simulink model "gnc"  (R2023b)
settings: Solver=VariableStepAuto  StartTime=0.0  StopTime=10.0  RelTol=1e-3
settings Model: DataDictionary=gnc_private.sldd  EnableAccessToBaseWorkspace=off  Creator=Miguel  LastModifiedBy=Miguel

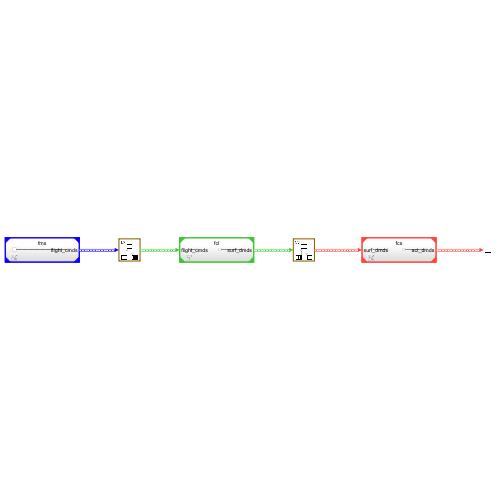
[thumbnail: Simulink's stored preview of the top-level diagram]
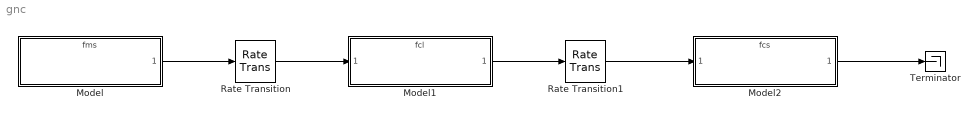
== system gnc ==
  Model : ModelReference  ModelNameDialog=fms.slx  SimulationMode=Normal  ModelReferenceVersion=1.11
  Model1 : ModelReference  ModelNameDialog=fcl.slx  SimulationMode=Normal  ModelReferenceVersion=1.12
  Model2 : ModelReference  ModelNameDialog=fcs.slx  SimulationMode=Normal  ModelReferenceVersion=1.12
  Rate Transition : RateTransition
  Rate Transition1 : RateTransition
  Terminator : Terminator
  wires:
  Model/1 -> Rate Transition/1
  Model1/1 -> Rate Transition1/1
  Model2/1 -> Terminator/1
  Rate Transition/1 -> Model1/1
  Rate Transition1/1 -> Model2/1
